simulink model "Reed_Solomon_Simulation"  (R2023a)
settings: Solver=VariableStepAuto  StartTime=0.0  StopTime=1000  RelTol=1e-3
undefined symbols (not defined in the file): rsgenpoly
libraries: commblkcod2 x2, commrandsrc3 x1
settings Model: Creator=caotr  LastModifiedBy=caotr

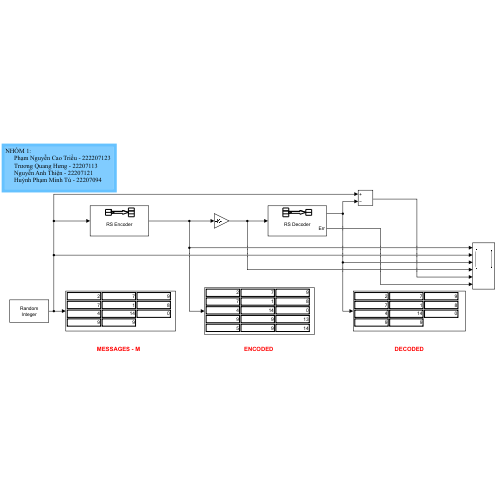
[thumbnail: Simulink's stored preview of the top-level diagram]
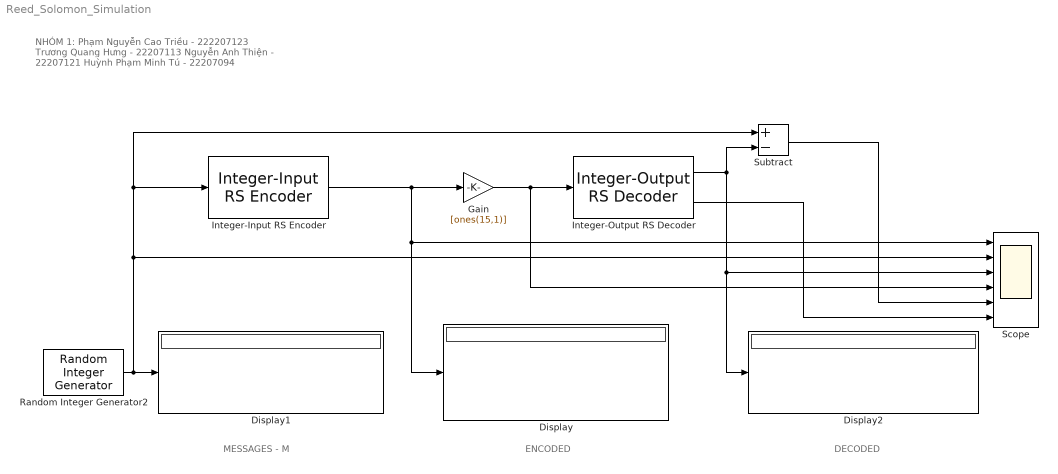
== system Reed_Solomon_Simulation ==
  note: MESSAGES - M
  note: NHÓM 1:
      | Phạm Nguyễn Cao Triều - 222207123
      | Trương Quang Hưng - 22207113
      | Nguyễn Anh Thiện - 22207121
      | Huỳnh Phạm Minh Tú - 22207094
  note: ENCODED
  note: DECODED
  Display : Display
  Display1 : Display
  Display2 : Display
  Gain : Gain  Gain=[ones(15,1)]
  Integer-Input RS Encoder : commblkcod2/Integer-Input RS Encoder  n=15  k=11  specShortening=off  shortenedK=3  specGenPoly=off  genPoly=rsgenpoly(7, 3, [], [], 'double')  specPrimPoly=off  prPoly='X^3 + X + 1'  specPuncture=off  punctVec=[ones(2,1); zeros(2,1)]
  Integer-Output RS Decoder : commblkcod2/Integer-Output RS Decoder  n=15  k=11  specShortening=off  shortenedK=3  specGenPoly=off  genPoly=rsgenpoly(7, 3, [], [], 'double')  specPrimPoly=off  prPoly='X^3 + X + 1'  specPuncture=off  punctVec=[ones(2,1); zeros(2,1)]  specErasurePort=off  showNumErr=on
  Random Integer Generator2 : commrandsrc3/Random Integer Generator  SetSize=15  SeedSource=Parameter  Seed=68521  SampleTime=1  SamplesPerFrame=11  OutputDataType=double  SimulateUsing=Interpreted execution
  Scope : Scope  NumInputPorts=6
  Subtract : Sum  Inputs=+-
  wires:
  Random Integer Generator2/1 -> Subtract/1, Integer-Input RS Encoder/1, Scope/2, Display1/1
  Integer-Input RS Encoder/1 -> Gain/1, Scope/1, Display/1
  Integer-Output RS Decoder/1 -> Scope/3, Display2/1, Subtract/2
  Integer-Output RS Decoder/2 -> Scope/6
  Subtract/1 -> Scope/5
  Gain/1 -> Integer-Output RS Decoder/1, Scope/4
